simulink model "Task2"  (R2024a)
settings: Solver=VariableStepAuto  StartTime=0.0  StopTime=100.0  RelTol=1e-3
settings Model: Creator=artemzmailov  LastModifiedBy=artemzmailov
settings DebuggingCC: IgnoredZcDiagnostic=none

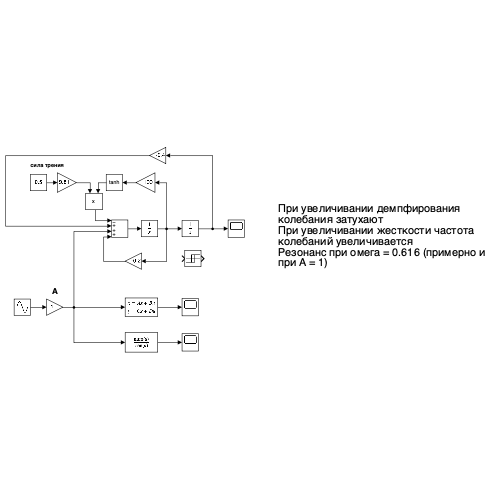
[thumbnail: Simulink's stored preview of the top-level diagram]
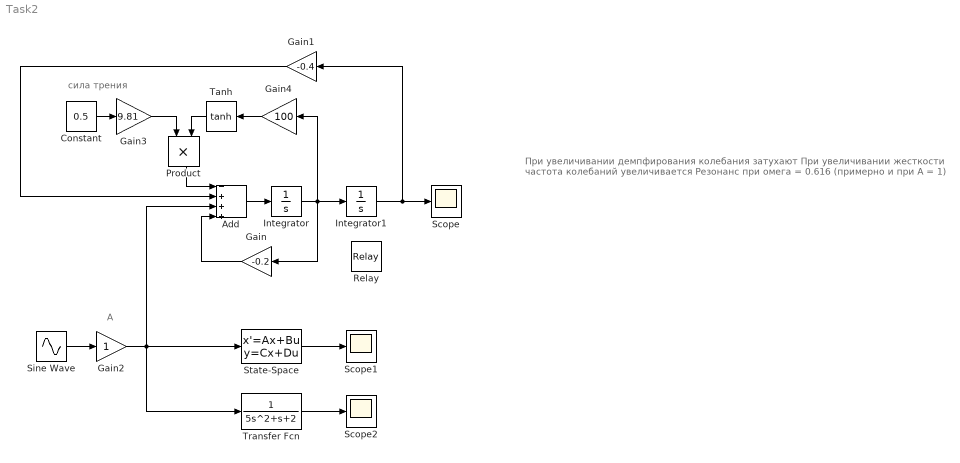
== system Task2 ==
  note: При увеличивании демпфирования колебания затухают
      | При увеличивании жесткости частота колебаний увеличивается
      | Резонанс при омега = 0.616 (примерно и при A = 1)
  note: сила трения
  note: А
  Add : Sum  Inputs=-+++
  Constant : Constant  Value=0.5
  Gain : Gain  Gain=-0.2
  Gain1 : Gain  Gain=-0.4
  Gain2 : Gain
  Gain3 : Gain  Gain=9.81
  Gain4 : Gain  Gain=100
  Integrator : Integrator
  Integrator1 : Integrator
  Product : Product
  Relay : Relay
  Scope : Scope
  Scope1 : Scope
  Scope2 : Scope
  Sine Wave : Sin  Amplitude=5  SampleTime=0
  State-Space : StateSpace  A=[0 1; -0.4 -0.2]  B=[0; 0.2]  C=[1, 0]  D=0  InitialCondition=0
  Tanh : Trigonometry  Operator=tanh
  Transfer Fcn : TransferFcn  Denominator=[5 1 2]
  wires:
  Integrator/1 -> Gain4/1, Gain/1, Integrator1/1
  Integrator1/1 -> Scope/1, Gain1/1
  Sine Wave/1 -> Gain2/1
  Add/1 -> Integrator/1
  State-Space/1 -> Scope1/1
  Transfer Fcn/1 -> Scope2/1
  Gain2/1 -> Add/3, State-Space/1, Transfer Fcn/1
  Gain/1 -> Add/4
  Constant/1 -> Gain3/1
  Gain1/1 -> Add/2
  Gain3/1 -> Product/1
  Product/1 -> Add/1
  Tanh/1 -> Product/2
  Gain4/1 -> Tanh/1
